simulink model "ROPOD_4Wheel_Tdistkinb_cntr_hosp_platform"  (R2017b)
settings: Solver=FixedStepAuto  StartTime=0.0  StopTime=Inf  FixedStep=Ts  RelTol=1e-3
PreLoadFcn:
  | init_model
InitFcn:
  | init_model
values from neighbouring files (symbols this model uses):
  FFtheta_intia = 0    [init_model.m]
  FFxy_mass = 0*80    (= 0)    [init_model.m]
  max_hw_tau = 7.0    (= 7)    [init_model.m]
  max_ropod_sw_force = 500    [init_model.m]
  max_ropod_sw_tau = 250    [init_model.m]
  Nwheels = 4    [Jqwl_numeric_function.m]    (also in S_matrix.m; extract_kinmodel_parameters.m; init_model.m; tau_optimal_dist_vec_fun.m)
  pivot_offs_sws = [2.663 3.74064 5.877 3.875]    [init_model.m]
  SW_COM1_ENABLE1 = hex2dec('0001')    [init_model.m]
  SW_COM1_ENABLE2 = hex2dec('0002')    [init_model.m]
  SW_COM1_MODE_TORQUE = bitshift(hex2dec('0000'),2)    [init_model.m]
  SW_COM1_MODE_VELOCITY = bitshift(hex2dec('0002'),2)    [init_model.m]
  SW_COM1_USE_TS = hex2dec('8000')    [init_model.m]
  sw_tau_2_curr = 1/motor_physical_parameters.torqueconstant.value    [init_model.m]
  Tinit = 5    [init_model.m]
  Ts = 0.001    [init_model.m]
  Tsp = 1    [init_model.m]
undefined symbols (not defined in the file or in its folder): DiscIntNeverNeededParam, Pose, ropod_kinmodel_param, Twist
libraries: robotlib x48, simulink x34, cstblocks x11, SOEM_EtherCAT_Lib x5, robotcorelib x1
(part 1 of 4)
PreSaveFcn:
  | init_model
settings Model: Creator=cesar  LastModifiedBy=cesar
settings OptimizationCC: PassReuseOutputArgsAs=Individual arguments  MaxStackSize=64
settings DebuggingCC: ParameterTunabilityLossMsg=error
settings HardwareCC: ProdBitPerLong=64  ProdHWDeviceType=Intel->x86-64 (Linux 64)  TargetBitPerLong=64  TargetBitPerPointer=64  TargetBitPerSizeT=64  TargetBitPerPtrDiffT=64  TargetLargestAtomicFloat=Float  TargetIntDivRoundTo=Zero  TargetEndianess=LittleEndian  TargetWordSize=64  TargetHWDeviceType=Intel->x86-64 (Linux 64)
settings SFSimCC: MATLABDynamicMemAlloc=off
settings RTWCC: SystemTargetFile=ert.tlc  HardwareBoard=Robot Operating System (ROS)  TemplateMakefile=ert_default_tmf  GenerateReport=on  RTWVerbose=off  CustomInclude=/usr/local/include/soem  CustomLibrary=/usr/local/lib/libsoem.so  Toolchain=Catkin  BuildConfiguration=Faster Runs  IncludeHyperlinkInReport=on  LaunchReport=on  TargetLang=C++  GenerateTraceInfo=on  GenerateTraceReport=on  GenerateTraceReportSl=on  GenerateTraceReportSf=on  GenerateTraceReportEml=on
settings CodeAppCC: ForceParamTrailComments=on  IgnoreCustomStorageClasses=off  OperatorAnnotations=on  SimulinkDataObjDesc=on  SFDataObjDesc=on  InsertBlockDesc=on
settings ERTTargetCC: SupportNonInlinedSFcns=on  SupportVariableSizeSignals=on

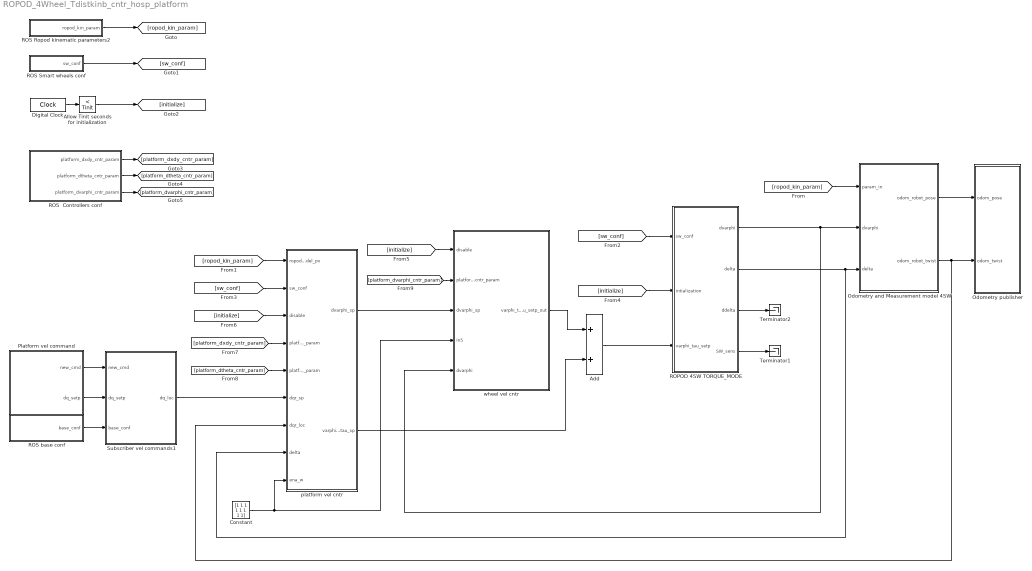
== system ROPOD_4Wheel_Tdistkinb_cntr_hosp_platform ==
  Add : Sum
  Allow Tinit seconds for initialization : simulink/Logic and Bit Operations/Compare To Constant  relop=<  const=Tinit  OutDataTypeStr=boolean
  Constant : Constant  Value=[1 1 1 1 1 1 1 1]
  Digital Clock : DigitalClock  SampleTime=Ts
  Odometry and Measurement model 4SW : Subsystem
  Odometry publisher : Subsystem
  Platform vel command : Subsystem
  ROPOD 4SW TORQUE_MODE : Subsystem
  ROS  Controllers conf : Subsystem
  ROS Ropod kinematic parameters2 : Subsystem
  ROS Smart wheels conf : Subsystem
  ROS base conf : Subsystem
  Subscriber vel commands1 : Subsystem
  Terminator1 : Terminator
  Terminator2 : Terminator
  platform vel cntr : Subsystem
  wheel vel cntr : Subsystem
  wires:
  Platform vel command/2(dq_setp) -> Subscriber vel commands1/2(dq_setp)
  ROS base conf/1(base_conf) -> Subscriber vel commands1/3(base_conf)
  ROPOD 4SW TORQUE_MODE/3(ddelta) -> Terminator2/1
  Add/1 -> ROPOD 4SW TORQUE_MODE/3(varphi_tau_setp)
  Constant/1 -> platform vel cntr/9(ena_w), wheel vel cntr/4(In5)
  Odometry and Measurement model 4SW/2(odom_robot_twist) -> platform vel cntr/7(dqr_loc), Odometry publisher/2(odom_twist)
  ROPOD 4SW TORQUE_MODE/4(SW_sens) -> Terminator1/1
  platform vel cntr/2(varphi_tau_sp) -> Add/2
  platform vel cntr/1(dvarphi_sp) -> wheel vel cntr/3(dvarphi_sp)
  ROPOD 4SW TORQUE_MODE/2(delta) -> platform vel cntr/8(delta), Odometry and Measurement model 4SW/3(delta)
  Digital Clock/1 -> Allow Tinit seconds for initialization/1
  ROS Ropod kinematic parameters2/1(ropod_kin_param) -> [ropod_kin_param]
  ROPOD 4SW TORQUE_MODE/1(dvarphi) -> Odometry and Measurement model 4SW/2(dvarphi), wheel vel cntr/5(dvarphi)
  ROS Smart wheels conf/1(sw_conf) -> [sw_conf]
  wheel vel cntr/1(varphi_tau_setp_out) -> Add/1
  Odometry and Measurement model 4SW/1(odom_robot_pose) -> Odometry publisher/1(odom_pose)
  Subscriber vel commands1/1(dq_loc) -> platform vel cntr/6(dqr_sp)
  [ropod_kin_param] -> Odometry and Measurement model 4SW/1(param_in)
  [ropod_kin_param] -> platform vel cntr/1(ropod_kinmodel_pv)
  [sw_conf] -> ROPOD 4SW TORQUE_MODE/1(sw_conf)
  [sw_conf] -> platform vel cntr/2(sw_conf)
  Allow Tinit seconds for initialization/1 -> [initialize]
  [initialize] -> ROPOD 4SW TORQUE_MODE/2(intialization)
  [initialize] -> wheel vel cntr/1(disable)
  [initialize] -> platform vel cntr/3(disable)
  ROS  Controllers conf/1(platform_dxdy_cntr_param) -> [platform_dxdy_cntr_param]
  ROS  Controllers conf/2(platform_dtheta_cntr_param) -> [platform_dtheta_cntr_param]
  ROS  Controllers conf/3(platform_dvarphi_cntr_param) -> [platform_dvarphi_cntr_param]
  [platform_dxdy_cntr_param] -> platform vel cntr/4(platform_dxdy_cntr_param)
  [platform_dtheta_cntr_param] -> platform vel cntr/5(platform_dtheta_cntr_param)
  [platform_dvarphi_cntr_param] -> wheel vel cntr/2(platform_dxdy_cntr_param)
  Platform vel command/1(new_cmd) -> Subscriber vel commands1/1(new_cmd)

== system ROPOD_4Wheel_Tdistkinb_cntr_hosp_platform/Odometry and Measurement model 4SW ==
  note: This output is only useful when using ros
      | This data is fed to /odom/pose
  note: This part is in global coordinates
  note: This part is in local coordinates
  param_in : Inport
  dvarphi : Inport  Port=2
  delta : Inport  Port=3
  Discrete-Time Integrator : DiscreteIntegrator  InitialConditionSetting=State (most efficient)  SampleTime=Ts  ICPrevOutput=DiscIntNeverNeededParam  ICPrevScaledInput=DiscIntNeverNeededParam
  Jqwl_matrix : MATLAB Function  TreatAsAtomicUnit=on
  Product3 : Product  Multiplication=Matrix(*)
  Selector3 : Selector  InputPortWidth=3  IndexOptions=Index vector (dialog)  Indices=3  OutputSizes=1
  Signal Specification : SignalSpecification  Dimensions=[3 1]
  pos_rot_matrix : MATLAB Function  TreatAsAtomicUnit=on
  odom_robot_pose : Outport
  odom_robot_twist : Outport  Port=2
  wires:
  Product3/1 -> Signal Specification/1
  param_in/1 -> Jqwl_matrix/1(ropod_kinmodel_param_vec)
  delta/1 -> Jqwl_matrix/2(delta)
  Jqwl_matrix/1(Jqwl) -> Product3/1
  dvarphi/1 -> Product3/2
  Signal Specification/1 -> pos_rot_matrix/1(dqr_loc), odom_robot_twist/1
  Selector3/1 -> pos_rot_matrix/2(theta_odom)
  pos_rot_matrix/1(dqr_glb) -> Discrete-Time Integrator/1
  Discrete-Time Integrator/1 -> odom_robot_pose/1, Selector3/1

== system ROPOD_4Wheel_Tdistkinb_cntr_hosp_platform/Odometry publisher ==
  odom_pose : Inport
  odom_twist : Inport  Port=2
  Blank Message : robotlib/Blank Message  SourceLibraryInfo=This block requires Robotics System Toolbox  messageType=nav_msgs/Odometry  SampleTime=-1
      settings: SourceProductBaseCode=RO
  Bus Assignment : BusAssignment  AssignedSignals=Pose.Pose.Position.X,Pose.Pose.Position.Y,Pose.Pose.Position.Z,Pose.Pose.Orientation.W,Pose.Pose.Orientation.X,Pose.Pose.Orientation.Y,Pose.Pose.Orientation.Z,Twist.Twist.Linear.X,Twist.Twist.Linear.Y,Twist.Twist.Linear.Z,Twist.Twist.Angular.X,Twist.Twist.Angular.Y,Twist.Twist.Angular.Z
  Constant{,1..5} (6 alike) : Constant  Value=0
  Coordinate Transformation Conversion : robotcorelib/Coordinate Transformation Conversion  InputRepresentation=Euler Angles  InputEulerSequence=XYZ  ShowTrVecInputPort=on  OutputRepresentation=Quaternion  OutputEulerSequence=ZYX  ShowTrVecOutputPort=on  SimulateUsing=Code generation
      settings: SourceProductBaseCode=RO
  Demux : Demux  Outputs=3
  Demux1 : Demux
  Demux2 : Demux  Outputs=3
  Mux : Mux  Inputs=3
  Publish : robotlib/Publish  SourceLibraryInfo=This block requires Robotics System Toolbox  topicSource=Specify your own  topic=/odom_incomplete  messageType=nav_msgs/Odometry  messageQueueLength=1
      settings: SourceProductBaseCode=RO
  Rate Transition : RateTransition  OutPortSampleTime=Ts_rost
  wires:
  Demux2/2 -> Bus Assignment/10
  Bus Assignment/1 -> Rate Transition/1
  Constant2/1 -> Mux/2
  Constant3/1 -> Bus Assignment/11
  Constant/1 -> Bus Assignment/4
  Constant4/1 -> Bus Assignment/12
  Demux2/1 -> Bus Assignment/9
  Coordinate Transformation Conversion/1 -> Demux1/1
  Constant5/1 -> Bus Assignment/13
  Demux/3 -> Mux/3
  Mux/1 -> Coordinate Transformation Conversion/1
  odom_pose/1 -> Demux/1
  Demux/1 -> Bus Assignment/2
  Constant1/1 -> Mux/1
  odom_twist/1 -> Demux2/1
  Demux/2 -> Bus Assignment/3
  Blank Message/1 -> Bus Assignment/1
  Demux2/3 -> Bus Assignment/14
  Rate Transition/1 -> Publish/1
  Demux1/1 -> Bus Assignment/5
  Demux1/2 -> Bus Assignment/6
  Demux1/3 -> Bus Assignment/7
  Demux1/4 -> Bus Assignment/8

== system ROPOD_4Wheel_Tdistkinb_cntr_hosp_platform/Platform vel command ==
  Subscribe1 : robotlib/Subscribe  SourceLibraryInfo=This block requires Robotics System Toolbox  topicSource=Specify your own  topic=/cmd_vel  messageType=geometry_msgs/Twist  sampleTime=Ts_rost  messageQueueLength=5
      settings: SourceProductBaseCode=RO
  new_cmd : Outport
  dq_setp : Outport  Port=2
  wires:
  Subscribe1/2 -> dq_setp/1
  Subscribe1/1 -> new_cmd/1

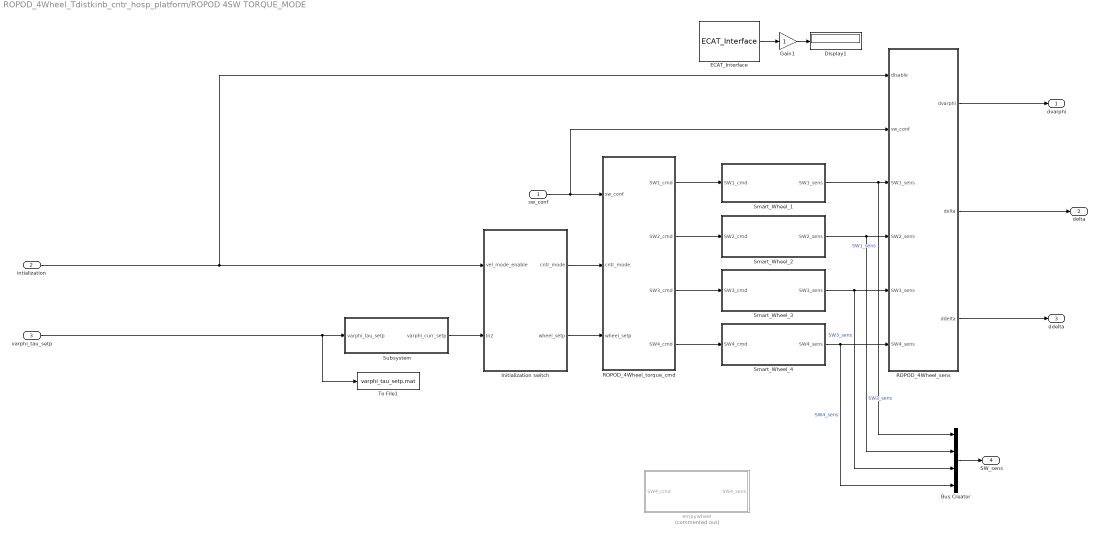
== system ROPOD_4Wheel_Tdistkinb_cntr_hosp_platform/ROPOD 4SW TORQUE_MODE ==
  sw_conf : Inport
  intialization : Inport  Port=2
  varphi_tau_setp : Inport  Port=3
  Bus Creator : BusCreator  Inputs=4
  Display1 : Display
  ECAT_Interface : SOEM_EtherCAT_Lib/ECAT_Interface  Priority=0  IFINTERFACE=eth0  TS=Ts
      settings: SourceProductName=SOEM_EtherCAT_Lib
  Gain1 : Gain  OutDataTypeStr=double
  Initialization switch : Subsystem
  ROPOD_4Wheel_sens : Subsystem
  ROPOD_4Wheel_torque_cmd : Subsystem
  Smart_Wheel_1 : Subsystem
  Smart_Wheel_2 : Subsystem
  Smart_Wheel_3 : Subsystem
  Smart_Wheel_4 : Subsystem
  Subsystem : Subsystem
  To File1 : ToFile  Filename=varphi_tau_setp.mat  MatrixName=varphi_tau_setp
  empywheel : Subsystem  Commented=on
  dvarphi : Outport
  delta : Outport  Port=2
  ddelta : Outport  Port=3
  SW_sens : Outport  Port=4
  wires:
  ROPOD_4Wheel_sens/2(delta) -> delta/1
  ROPOD_4Wheel_sens/1(dvarphi) -> dvarphi/1
  ECAT_Interface/1 -> Gain1/1
  Gain1/1 -> Display1/1
  ROPOD_4Wheel_sens/3(ddelta) -> ddelta/1
  ROPOD_4Wheel_torque_cmd/4(SW4_cmd) -> Smart_Wheel_4/1(SW4_cmd)
  ROPOD_4Wheel_torque_cmd/1(SW1_cmd) -> Smart_Wheel_1/1(SW1_cmd)
  ROPOD_4Wheel_torque_cmd/3(SW3_cmd) -> Smart_Wheel_3/1(SW3_cmd)
  sw_conf/1 -> ROPOD_4Wheel_torque_cmd/1(sw_conf), ROPOD_4Wheel_sens/2(sw_conf)
  ROPOD_4Wheel_torque_cmd/2(SW2_cmd) -> Smart_Wheel_2/1(SW2_cmd)
  Smart_Wheel_1/1(SW1_sens) -> Bus Creator/1, ROPOD_4Wheel_sens/3(SW1_sens)  "SW1_sens"
  Smart_Wheel_4/1(SW4_sens) -> ROPOD_4Wheel_sens/6(SW4_sens), Bus Creator/4  "SW4_sens"
  Smart_Wheel_2/1(SW2_sens) -> ROPOD_4Wheel_sens/4(SW2_sens), Bus Creator/2  "SW2_sens"
  Smart_Wheel_3/1(SW3_sens) -> ROPOD_4Wheel_sens/5(SW3_sens), Bus Creator/3  "SW3_sens"
  Bus Creator/1 -> SW_sens/1
  Initialization switch/1(cntr_mode) -> ROPOD_4Wheel_torque_cmd/2(cntr_mode)
  Initialization switch/2(wheel_setp) -> ROPOD_4Wheel_torque_cmd/3(wheel_setp)
  Subsystem/1(varphi_curr_setp) -> Initialization switch/2(In2)
  varphi_tau_setp/1 -> To File1/1, Subsystem/1(varphi_tau_setp)
  intialization/1 -> ROPOD_4Wheel_sens/1(disable), Initialization switch/1(vel_mode_enable)

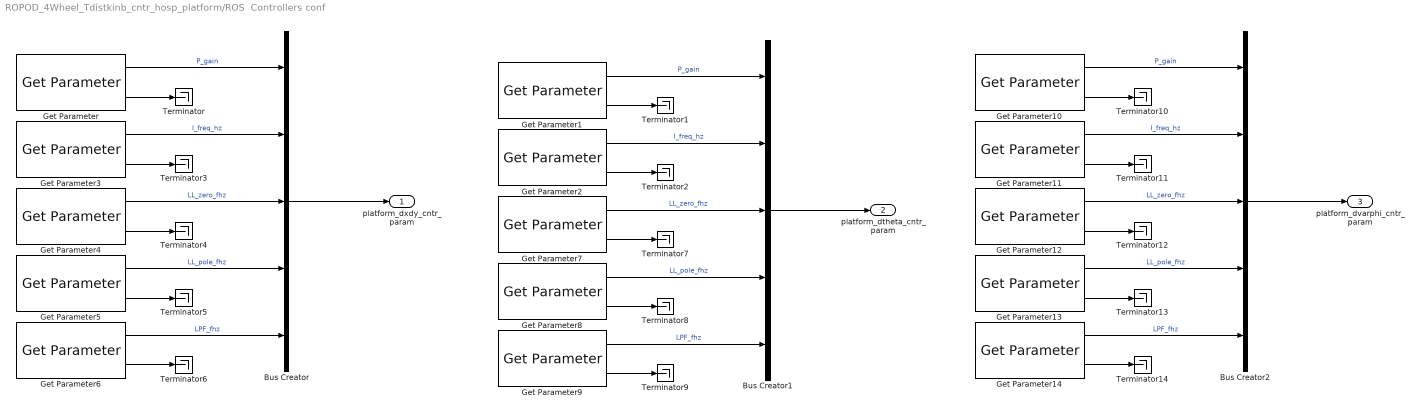
== system ROPOD_4Wheel_Tdistkinb_cntr_hosp_platform/ROS  Controllers conf ==
  Bus Creator : BusCreator  Inputs=5
  Bus Creator1 : BusCreator  Inputs=5
  Bus Creator2 : BusCreator  Inputs=5
  Get Parameter : robotlib/Get Parameter  SourceLibraryInfo=This block requires Robotics System Toolbox  ParameterSource=Specify your own  ParameterName=/ropod/ropod_4wheel_kinb_cntr_node/platform_dxdy_cntr/Kgain  ParameterType=double  ParameterMaxArrayLength=16  ParameterInitialValue=K_gain_dxdy_cntr  SampleTime=Tsp  ShowErrorCodeOutput=on  ModelName=ROPOD_4Wheel_Tdistkinb_cntr  BlockId=ParamGet_ROPOD_4Wheel_Tdistkinb_cntr_2716
      settings: SourceProductName=Robotics System Toolbox  SourceProductBaseCode=RO
  Get Parameter1 : robotlib/Get Parameter  SourceLibraryInfo=This block requires Robotics System Toolbox  ParameterSource=Specify your own  ParameterName=/ropod/ropod_4wheel_kinb_cntr_node/platform_dtheta_cntr/Kgain  ParameterType=double  ParameterMaxArrayLength=16  ParameterInitialValue=K_gain_dtheta_cntr  SampleTime=Tsp  ShowErrorCodeOutput=on  ModelName=ROPOD_4Wheel_Tdistkinb_cntr  BlockId=ParamGet_ROPOD_4Wheel_Tdistkinb_cntr_2919
      settings: SourceProductName=Robotics System Toolbox  SourceProductBaseCode=RO
  Get Parameter10 : robotlib/Get Parameter  SourceLibraryInfo=This block requires Robotics System Toolbox  ParameterSource=Specify your own  ParameterName=/ropod/ropod_4wheel_kinb_cntr_node/platform_dvarphi_cntr/Kgain  ParameterType=double  ParameterMaxArrayLength=16  ParameterInitialValue=K_gain_dvarphi_cntr  SampleTime=Tsp  ShowErrorCodeOutput=on  ModelName=ROPOD_4Wheel_Tdistkinb_cntr  BlockId=ParamGet_ROPOD_4Wheel_Tdistkinb_cntr_2931
      settings: SourceProductName=Robotics System Toolbox  SourceProductBaseCode=RO
  Get Parameter11 : robotlib/Get Parameter  SourceLibraryInfo=This block requires Robotics System Toolbox  ParameterSource=Specify your own  ParameterName=/ropod/ropod_4wheel_kinb_cntr_node/platform_dvarphi_cntr/I_fhz  ParameterType=double  ParameterMaxArrayLength=16  ParameterInitialValue=I_fhz_dvarphi_cntr  SampleTime=Tsp  ShowErrorCodeOutput=on  ModelName=ROPOD_4Wheel_Tdistkinb_cntr  BlockId=ParamGet_ROPOD_4Wheel_Tdistkinb_cntr_2932
      settings: SourceProductName=Robotics System Toolbox  SourceProductBaseCode=RO
  Get Parameter12 : robotlib/Get Parameter  SourceLibraryInfo=This block requires Robotics System Toolbox  ParameterSource=Specify your own  ParameterName=/ropod/ropod_4wheel_kinb_cntr_node/platform_dvarphi_cntr/LL_wz_fhz  ParameterType=double  ParameterMaxArrayLength=16  ParameterInitialValue=LL_wz_fhz_dvarphi_cntr  SampleTime=Tsp  ShowErrorCodeOutput=on  ModelName=ROPOD_4Wheel_Tdistkinb_cntr  BlockId=ParamGet_ROPOD_4Wheel_Tdistkinb_cntr_2933
      settings: SourceProductName=Robotics System Toolbox  SourceProductBaseCode=RO
  Get Parameter13 : robotlib/Get Parameter  SourceLibraryInfo=This block requires Robotics System Toolbox  ParameterSource=Specify your own  ParameterName=/ropod/ropod_4wheel_kinb_cntr_node/platform_dvarphi_cntr/LL_wp_fhz  ParameterType=double  ParameterMaxArrayLength=16  ParameterInitialValue=LL_wp_fhz_dvarphi_cntr  SampleTime=Tsp  ShowErrorCodeOutput=on  ModelName=ROPOD_4Wheel_Tdistkinb_cntr  BlockId=ParamGet_ROPOD_4Wheel_Tdistkinb_cntr_2934
      settings: SourceProductName=Robotics System Toolbox  SourceProductBaseCode=RO
  Get Parameter14 : robotlib/Get Parameter  SourceLibraryInfo=This block requires Robotics System Toolbox  ParameterSource=Specify your own  ParameterName=/ropod/ropod_4wheel_kinb_cntr_node/platform_dvarphi_cntr/LPF_fhz  ParameterType=double  ParameterMaxArrayLength=16  ParameterInitialValue=LPF_fhz_dvarphi_cntr  SampleTime=Tsp  ShowErrorCodeOutput=on  ModelName=ROPOD_4Wheel_Tdistkinb_cntr  BlockId=ParamGet_ROPOD_4Wheel_Tdistkinb_cntr_2935
      settings: SourceProductName=Robotics System Toolbox  SourceProductBaseCode=RO
  Get Parameter2 : robotlib/Get Parameter  SourceLibraryInfo=This block requires Robotics System Toolbox  ParameterSource=Specify your own  ParameterName=/ropod/ropod_4wheel_kinb_cntr_node/platform_dtheta_cntr/I_fhz  ParameterType=double  ParameterMaxArrayLength=16  ParameterInitialValue=I_fhz_dtheta_cntr  SampleTime=Tsp  ShowErrorCodeOutput=on  ModelName=ROPOD_4Wheel_Tdistkinb_cntr  BlockId=ParamGet_ROPOD_4Wheel_Tdistkinb_cntr_2920
      settings: SourceProductName=Robotics System Toolbox  SourceProductBaseCode=RO
  Get Parameter3 : robotlib/Get Parameter  SourceLibraryInfo=This block requires Robotics System Toolbox  ParameterSource=Specify your own  ParameterName=/ropod/ropod_4wheel_kinb_cntr_node/platform_dxdy_cntr/I_fhz  ParameterType=double  ParameterMaxArrayLength=16  ParameterInitialValue=I_fhz_dxdy_cntr  SampleTime=Tsp  ShowErrorCodeOutput=on  ModelName=ROPOD_4Wheel_Tdistkinb_cntr  BlockId=ParamGet_ROPOD_4Wheel_Tdistkinb_cntr_2898
      settings: SourceProductName=Robotics System Toolbox  SourceProductBaseCode=RO
  Get Parameter4 : robotlib/Get Parameter  SourceLibraryInfo=This block requires Robotics System Toolbox  ParameterSource=Specify your own  ParameterName=/ropod/ropod_4wheel_kinb_cntr_node/platform_dxdy_cntr/LL_wz_fhz  ParameterType=double  ParameterMaxArrayLength=16  ParameterInitialValue=LL_wz_fhz_dxdy_cntr  SampleTime=Tsp  ShowErrorCodeOutput=on  ModelName=ROPOD_4Wheel_Tdistkinb_cntr  BlockId=ParamGet_ROPOD_4Wheel_Tdistkinb_cntr_2900
      settings: SourceProductName=Robotics System Toolbox  SourceProductBaseCode=RO
  Get Parameter5 : robotlib/Get Parameter  SourceLibraryInfo=This block requires Robotics System Toolbox  ParameterSource=Specify your own  ParameterName=/ropod/ropod_4wheel_kinb_cntr_node/platform_dxdy_cntr/LL_wp_fhz  ParameterType=double  ParameterMaxArrayLength=16  ParameterInitialValue=LL_wp_fhz_dxdy_cntr  SampleTime=Tsp  ShowErrorCodeOutput=on  ModelName=ROPOD_4Wheel_Tdistkinb_cntr  BlockId=ParamGet_ROPOD_4Wheel_Tdistkinb_cntr_2902
      settings: SourceProductName=Robotics System Toolbox  SourceProductBaseCode=RO
  Get Parameter6 : robotlib/Get Parameter  SourceLibraryInfo=This block requires Robotics System Toolbox  ParameterSource=Specify your own  ParameterName=/ropod/ropod_4wheel_kinb_cntr_node/platform_dxdy_cntr/LPF_fhz  ParameterType=double  ParameterMaxArrayLength=16  ParameterInitialValue=LPF_fhz_dxdy_cntr  SampleTime=Tsp  ShowErrorCodeOutput=on  ModelName=ROPOD_4Wheel_Tdistkinb_cntr  BlockId=ParamGet_ROPOD_4Wheel_Tdistkinb_cntr_2903
      settings: SourceProductName=Robotics System Toolbox  SourceProductBaseCode=RO
  Get Parameter7 : robotlib/Get Parameter  SourceLibraryInfo=This block requires Robotics System Toolbox  ParameterSource=Specify your own  ParameterName=/ropod/ropod_4wheel_kinb_cntr_node/platform_dtheta_cntr/LL_wz_fhz  ParameterType=double  ParameterMaxArrayLength=16  ParameterInitialValue=LL_wz_fhz_dtheta_cntr  SampleTime=Tsp  ShowErrorCodeOutput=on  ModelName=ROPOD_4Wheel_Tdistkinb_cntr  BlockId=ParamGet_ROPOD_4Wheel_Tdistkinb_cntr_2921
      settings: SourceProductName=Robotics System Toolbox  SourceProductBaseCode=RO
  Get Parameter8 : robotlib/Get Parameter  SourceLibraryInfo=This block requires Robotics System Toolbox  ParameterSource=Specify your own  ParameterName=/ropod/ropod_4wheel_kinb_cntr_node/platform_dtheta_cntr/LL_wp_fhz  ParameterType=double  ParameterMaxArrayLength=16  ParameterInitialValue=LL_wp_fhz_dtheta_cntr  SampleTime=Tsp  ShowErrorCodeOutput=on  ModelName=ROPOD_4Wheel_Tdistkinb_cntr  BlockId=ParamGet_ROPOD_4Wheel_Tdistkinb_cntr_2922
      settings: SourceProductName=Robotics System Toolbox  SourceProductBaseCode=RO
  Get Parameter9 : robotlib/Get Parameter  SourceLibraryInfo=This block requires Robotics System Toolbox  ParameterSource=Specify your own  ParameterName=/ropod/ropod_4wheel_kinb_cntr_node/platform_dtheta_cntr/LPF_fhz  ParameterType=double  ParameterMaxArrayLength=16  ParameterInitialValue=LPF_fhz_dtheta_cntr  SampleTime=Tsp  ShowErrorCodeOutput=on  ModelName=ROPOD_4Wheel_Tdistkinb_cntr  BlockId=ParamGet_ROPOD_4Wheel_Tdistkinb_cntr_2923
      settings: SourceProductName=Robotics System Toolbox  SourceProductBaseCode=RO
  Terminator{,1..14} (15 alike) : Terminator
  platform_dxdy_cntr_param : Outport
  platform_dtheta_cntr_param : Outport  Port=2
  platform_dvarphi_cntr_param : Outport  Port=3
  wires:
  Get Parameter/2 -> Terminator/1
  Get Parameter5/1 -> Bus Creator/4  "LL_pole_fhz"
  Get Parameter6/1 -> Bus Creator/5  "LPF_fhz"
  Bus Creator/1 -> platform_dxdy_cntr_param/1
  Get Parameter3/1 -> Bus Creator/2  "I_freq_hz"
  Get Parameter4/1 -> Bus Creator/3  "LL_zero_fhz"
  Get Parameter/1 -> Bus Creator/1  "P_gain"
  Get Parameter3/2 -> Terminator3/1
  Get Parameter4/2 -> Terminator4/1
  Get Parameter5/2 -> Terminator5/1
  Get Parameter6/2 -> Terminator6/1
  Get Parameter8/1 -> Bus Creator1/4  "LL_pole_fhz"
  Get Parameter9/2 -> Terminator9/1
  Get Parameter2/1 -> Bus Creator1/2  "I_freq_hz"
  Get Parameter8/2 -> Terminator8/1
  Bus Creator1/1 -> platform_dtheta_cntr_param/1
  Get Parameter2/2 -> Terminator2/1
  Get Parameter7/1 -> Bus Creator1/3  "LL_zero_fhz"
  Get Parameter7/2 -> Terminator7/1
  Get Parameter1/1 -> Bus Creator1/1  "P_gain"
  Get Parameter1/2 -> Terminator1/1
  Get Parameter9/1 -> Bus Creator1/5  "LPF_fhz"
  Get Parameter10/2 -> Terminator10/1
  Get Parameter13/2 -> Terminator13/1
  Get Parameter14/2 -> Terminator14/1
  Get Parameter11/1 -> Bus Creator2/2  "I_freq_hz"
  Get Parameter10/1 -> Bus Creator2/1  "P_gain"
  Get Parameter11/2 -> Terminator11/1
  Get Parameter13/1 -> Bus Creator2/4  "LL_pole_fhz"
  Bus Creator2/1 -> platform_dvarphi_cntr_param/1
  Get Parameter12/2 -> Terminator12/1
  Get Parameter12/1 -> Bus Creator2/3  "LL_zero_fhz"
  Get Parameter14/1 -> Bus Creator2/5  "LPF_fhz"

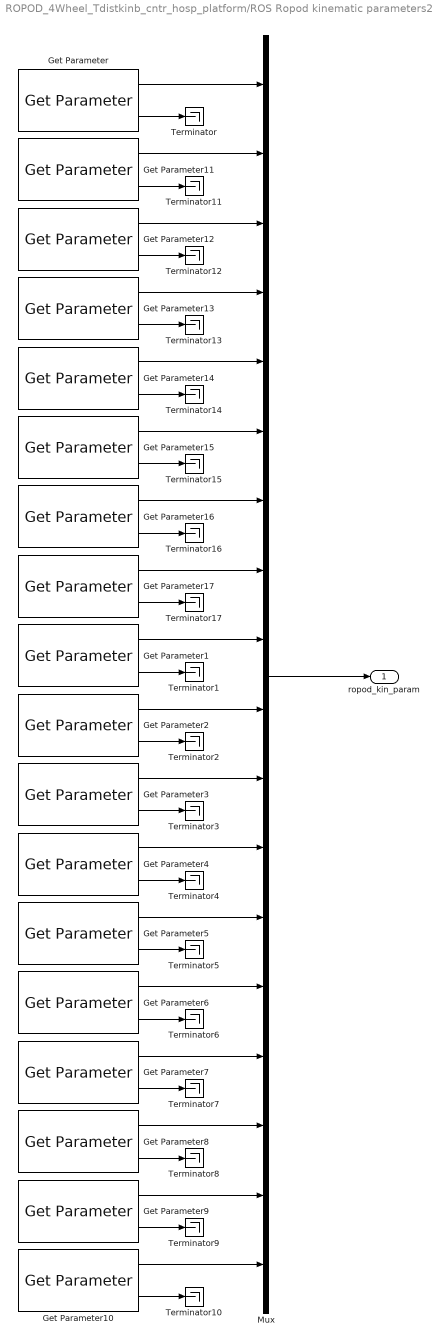
== system ROPOD_4Wheel_Tdistkinb_cntr_hosp_platform/ROS Ropod kinematic parameters2 ==
  Get Parameter : robotlib/Get Parameter  SourceLibraryInfo=This block requires Robotics System Toolbox  ParameterSource=Specify your own  ParameterName=/ropod/ropod_4wheel_kinb_cntr_node/base_kin_model/r_wL_SW1  ParameterType=double  ParameterMaxArrayLength=16  ParameterInitialValue=ropod_kinmodel_param.r_w(1)  SampleTime=Tsp  ShowErrorCodeOutput=on  ModelName=ROPOD_4Wheel_Tdistkinb_cntr  BlockId=ParamGet_ROPOD_4Wheel_Tdistkinb_cntr_2173
      settings: SourceProductName=Robotics System Toolbox  SourceProductBaseCode=RO
  Get Parameter1 : robotlib/Get Parameter  SourceLibraryInfo=This block requires Robotics System Toolbox  ParameterSource=Specify your own  ParameterName=/ropod/ropod_4wheel_kinb_cntr_node/base_kin_model/s_w  ParameterType=double  ParameterMaxArrayLength=16  ParameterInitialValue=ropod_kinmodel_param.s_w  SampleTime=Tsp  ShowErrorCodeOutput=on  ModelName=ROPOD_4Wheel_Tdistkinb_cntr  BlockId=ParamGet_ROPOD_4Wheel_Tdistkinb_cntr_2174
      settings: SourceProductName=Robotics System Toolbox  SourceProductBaseCode=RO
  Get Parameter10 : robotlib/Get Parameter  SourceLibraryInfo=This block requires Robotics System Toolbox  ParameterSource=Specify your own  ParameterName=/ropod/ropod_4wheel_kinb_cntr_node/base_kin_model/ypos_SW4  ParameterType=double  ParameterMaxArrayLength=16  ParameterInitialValue=ropod_kinmodel_param.C_SW(8)  SampleTime=Tsp  ShowErrorCodeOutput=on  ModelName=ROPOD_4Wheel_Tdistkinb_cntr  BlockId=ParamGet_ROPOD_4Wheel_Tdistkinb_cntr_2175
      settings: SourceProductName=Robotics System Toolbox  SourceProductBaseCode=RO
  Get Parameter11 : robotlib/Get Parameter  SourceLibraryInfo=This block requires Robotics System Toolbox  ParameterSource=Specify your own  ParameterName=/ropod/ropod_4wheel_kinb_cntr_node/base_kin_model/r_wR_SW1  ParameterType=double  ParameterMaxArrayLength=16  ParameterInitialValue=ropod_kinmodel_param.r_w(2)  SampleTime=Tsp  ShowErrorCodeOutput=on  ModelName=ROPOD_4Wheel_Tdistkinb_cntr  BlockId=ParamGet_ROPOD_4Wheel_Tdistkinb_cntr_2176
      settings: SourceProductName=Robotics System Toolbox  SourceProductBaseCode=RO
  Get Parameter12 : robotlib/Get Parameter  SourceLibraryInfo=This block requires Robotics System Toolbox  ParameterSource=Specify your own  ParameterName=/ropod/ropod_4wheel_kinb_cntr_node/base_kin_model/r_wL_SW2  ParameterType=double  ParameterMaxArrayLength=16  ParameterInitialValue=ropod_kinmodel_param.r_w(3)  SampleTime=Tsp  ShowErrorCodeOutput=on  ModelName=ROPOD_4Wheel_Tdistkinb_cntr  BlockId=ParamGet_ROPOD_4Wheel_Tdistkinb_cntr_2177
      settings: SourceProductName=Robotics System Toolbox  SourceProductBaseCode=RO
  Get Parameter13 : robotlib/Get Parameter  SourceLibraryInfo=This block requires Robotics System Toolbox  ParameterSource=Specify your own  ParameterName=/ropod/ropod_4wheel_kinb_cntr_node/base_kin_model/r_wR_SW2  ParameterType=double  ParameterMaxArrayLength=16  ParameterInitialValue=ropod_kinmodel_param.r_w(4)  SampleTime=Tsp  ShowErrorCodeOutput=on  ModelName=ROPOD_4Wheel_Tdistkinb_cntr  BlockId=ParamGet_ROPOD_4Wheel_Tdistkinb_cntr_2178
      settings: SourceProductName=Robotics System Toolbox  SourceProductBaseCode=RO
  Get Parameter14 : robotlib/Get Parameter  SourceLibraryInfo=This block requires Robotics System Toolbox  ParameterSource=Specify your own  ParameterName=/ropod/ropod_4wheel_kinb_cntr_node/base_kin_model/r_wL_SW3  ParameterType=double  ParameterMaxArrayLength=16  ParameterInitialValue=ropod_kinmodel_param.r_w(5)  SampleTime=Tsp  ShowErrorCodeOutput=on  ModelName=ROPOD_4Wheel_Tdistkinb_cntr  BlockId=ParamGet_ROPOD_4Wheel_Tdistkinb_cntr_2179
      settings: SourceProductName=Robotics System Toolbox  SourceProductBaseCode=RO
  Get Parameter15 : robotlib/Get Parameter  SourceLibraryInfo=This block requires Robotics System Toolbox  ParameterSource=Specify your own  ParameterName=/ropod/ropod_4wheel_kinb_cntr_node/base_kin_model/r_wR_SW3  ParameterType=double  ParameterMaxArrayLength=16  ParameterInitialValue=ropod_kinmodel_param.r_w(6)  SampleTime=Tsp  ShowErrorCodeOutput=on  ModelName=ROPOD_4Wheel_Tdistkinb_cntr  BlockId=ParamGet_ROPOD_4Wheel_Tdistkinb_cntr_2180
      settings: SourceProductName=Robotics System Toolbox  SourceProductBaseCode=RO
  Get Parameter16 : robotlib/Get Parameter  SourceLibraryInfo=This block requires Robotics System Toolbox  ParameterSource=Specify your own  ParameterName=/ropod/ropod_4wheel_kinb_cntr_node/base_kin_model/r_wL_SW4  ParameterType=double  ParameterMaxArrayLength=16  ParameterInitialValue=ropod_kinmodel_param.r_w(7)  SampleTime=Tsp  ShowErrorCodeOutput=on  ModelName=ROPOD_4Wheel_Tdistkinb_cntr  BlockId=ParamGet_ROPOD_4Wheel_Tdistkinb_cntr_2181
      settings: SourceProductName=Robotics System Toolbox  SourceProductBaseCode=RO
  Get Parameter17 : robotlib/Get Parameter  SourceLibraryInfo=This block requires Robotics System Toolbox  ParameterSource=Specify your own  ParameterName=/ropod/ropod_4wheel_kinb_cntr_node/base_kin_model/r_wR_SW4  ParameterType=double  ParameterMaxArrayLength=16  ParameterInitialValue=ropod_kinmodel_param.r_w(8)  SampleTime=Tsp  ShowErrorCodeOutput=on  ModelName=ROPOD_4Wheel_Tdistkinb_cntr  BlockId=ParamGet_ROPOD_4Wheel_Tdistkinb_cntr_2182
      settings: SourceProductName=Robotics System Toolbox  SourceProductBaseCode=RO
  Get Parameter2 : robotlib/Get Parameter  SourceLibraryInfo=This block requires Robotics System Toolbox  ParameterSource=Specify your own  ParameterName=/ropod/ropod_4wheel_kinb_cntr_node/base_kin_model/d_w  ParameterType=double  ParameterMaxArrayLength=16  ParameterInitialValue=ropod_kinmodel_param.d_w  SampleTime=Tsp  ShowErrorCodeOutput=on  ModelName=ROPOD_4Wheel_Tdistkinb_cntr  BlockId=ParamGet_ROPOD_4Wheel_Tdistkinb_cntr_2183
      settings: SourceProductName=Robotics System Toolbox  SourceProductBaseCode=RO
  Get Parameter3 : robotlib/Get Parameter  SourceLibraryInfo=This block requires Robotics System Toolbox  ParameterSource=Specify your own  ParameterName=/ropod/ropod_4wheel_kinb_cntr_node/base_kin_model/xpos_SW1  ParameterType=double  ParameterMaxArrayLength=16  ParameterInitialValue=ropod_kinmodel_param.C_SW(1)  SampleTime=Tsp  ShowErrorCodeOutput=on  ModelName=ROPOD_4Wheel_Tdistkinb_cntr  BlockId=ParamGet_ROPOD_4Wheel_Tdistkinb_cntr_2184
      settings: SourceProductName=Robotics System Toolbox  SourceProductBaseCode=RO
  Get Parameter4 : robotlib/Get Parameter  SourceLibraryInfo=This block requires Robotics System Toolbox  ParameterSource=Specify your own  ParameterName=/ropod/ropod_4wheel_kinb_cntr_node/base_kin_model/ypos_SW1  ParameterType=double  ParameterMaxArrayLength=16  ParameterInitialValue=ropod_kinmodel_param.C_SW(2)  SampleTime=Tsp  ShowErrorCodeOutput=on  ModelName=ROPOD_4Wheel_Tdistkinb_cntr  BlockId=ParamGet_ROPOD_4Wheel_Tdistkinb_cntr_2185
      settings: SourceProductName=Robotics System Toolbox  SourceProductBaseCode=RO
  Get Parameter5 : robotlib/Get Parameter  SourceLibraryInfo=This block requires Robotics System Toolbox  ParameterSource=Specify your own  ParameterName=/ropod/ropod_4wheel_kinb_cntr_node/base_kin_model/xpos_SW2  ParameterType=double  ParameterMaxArrayLength=16  ParameterInitialValue=ropod_kinmodel_param.C_SW(3)  SampleTime=Tsp  ShowErrorCodeOutput=on  ModelName=ROPOD_4Wheel_Tdistkinb_cntr  BlockId=ParamGet_ROPOD_4Wheel_Tdistkinb_cntr_2186
      settings: SourceProductName=Robotics System Toolbox  SourceProductBaseCode=RO
  Get Parameter6 : robotlib/Get Parameter  SourceLibraryInfo=This block requires Robotics System Toolbox  ParameterSource=Specify your own  ParameterName=/ropod/ropod_4wheel_kinb_cntr_node/base_kin_model/ypos_SW2  ParameterType=double  ParameterMaxArrayLength=16  ParameterInitialValue=ropod_kinmodel_param.C_SW(4)  SampleTime=Tsp  ShowErrorCodeOutput=on  ModelName=ROPOD_4Wheel_Tdistkinb_cntr  BlockId=ParamGet_ROPOD_4Wheel_Tdistkinb_cntr_2187
      settings: SourceProductName=Robotics System Toolbox  SourceProductBaseCode=RO
  Get Parameter7 : robotlib/Get Parameter  SourceLibraryInfo=This block requires Robotics System Toolbox  ParameterSource=Specify your own  ParameterName=/ropod/ropod_4wheel_kinb_cntr_node/base_kin_model/xpos_SW3  ParameterType=double  ParameterMaxArrayLength=16  ParameterInitialValue=ropod_kinmodel_param.C_SW(5)  SampleTime=Tsp  ShowErrorCodeOutput=on  ModelName=ROPOD_4Wheel_Tdistkinb_cntr  BlockId=ParamGet_ROPOD_4Wheel_Tdistkinb_cntr_2188
      settings: SourceProductName=Robotics System Toolbox  SourceProductBaseCode=RO
  Get Parameter8 : robotlib/Get Parameter  SourceLibraryInfo=This block requires Robotics System Toolbox  ParameterSource=Specify your own  ParameterName=/ropod/ropod_4wheel_kinb_cntr_node/base_kin_model/ypos_SW3  ParameterType=double  ParameterMaxArrayLength=16  ParameterInitialValue=ropod_kinmodel_param.C_SW(6)  SampleTime=Tsp  ShowErrorCodeOutput=on  ModelName=ROPOD_4Wheel_Tdistkinb_cntr  BlockId=ParamGet_ROPOD_4Wheel_Tdistkinb_cntr_2189
      settings: SourceProductName=Robotics System Toolbox  SourceProductBaseCode=RO
  Get Parameter9 : robotlib/Get Parameter  SourceLibraryInfo=This block requires Robotics System Toolbox  ParameterSource=Specify your own  ParameterName=/ropod/ropod_4wheel_kinb_cntr_node/base_kin_model/xpos_SW4  ParameterType=double  ParameterMaxArrayLength=16  ParameterInitialValue=ropod_kinmodel_param.C_SW(7)  SampleTime=Tsp  ShowErrorCodeOutput=on  ModelName=ROPOD_4Wheel_Tdistkinb_cntr  BlockId=ParamGet_ROPOD_4Wheel_Tdistkinb_cntr_2190
      settings: SourceProductName=Robotics System Toolbox  SourceProductBaseCode=RO
  Mux : Mux  Inputs=18
  Terminator{,1..17} (18 alike) : Terminator
  ropod_kin_param : Outport
  wires:
  Mux/1 -> ropod_kin_param/1
  Get Parameter/2 -> Terminator/1
  Get Parameter13/1 -> Mux/4
  Get Parameter15/2 -> Terminator15/1
  Get Parameter14/2 -> Terminator14/1
  Get Parameter16/1 -> Mux/7
  Get Parameter15/1 -> Mux/6
  Get Parameter11/1 -> Mux/2
  Get Parameter11/2 -> Terminator11/1
  Get Parameter16/2 -> Terminator16/1
  Get Parameter12/2 -> Terminator12/1
  Get Parameter12/1 -> Mux/3
  Get Parameter/1 -> Mux/1
  Get Parameter17/2 -> Terminator17/1
  Get Parameter13/2 -> Terminator13/1
  Get Parameter17/1 -> Mux/8
  Get Parameter14/1 -> Mux/5
  Get Parameter2/2 -> Terminator2/1
  Get Parameter2/1 -> Mux/10
  Get Parameter1/1 -> Mux/9
  Get Parameter1/2 -> Terminator1/1
  Get Parameter6/2 -> Terminator6/1
  Get Parameter6/1 -> Mux/14
  Get Parameter3/1 -> Mux/11
  Get Parameter5/2 -> Terminator5/1
  Get Parameter5/1 -> Mux/13
  Get Parameter4/1 -> Mux/12
  Get Parameter3/2 -> Terminator3/1
  Get Parameter4/2 -> Terminator4/1
  Get Parameter10/1 -> Mux/18
  Get Parameter10/2 -> Terminator10/1
  Get Parameter8/2 -> Terminator8/1
  Get Parameter7/2 -> Terminator7/1
  Get Parameter9/2 -> Terminator9/1
  Get Parameter7/1 -> Mux/15
  Get Parameter8/1 -> Mux/16
  Get Parameter9/1 -> Mux/17

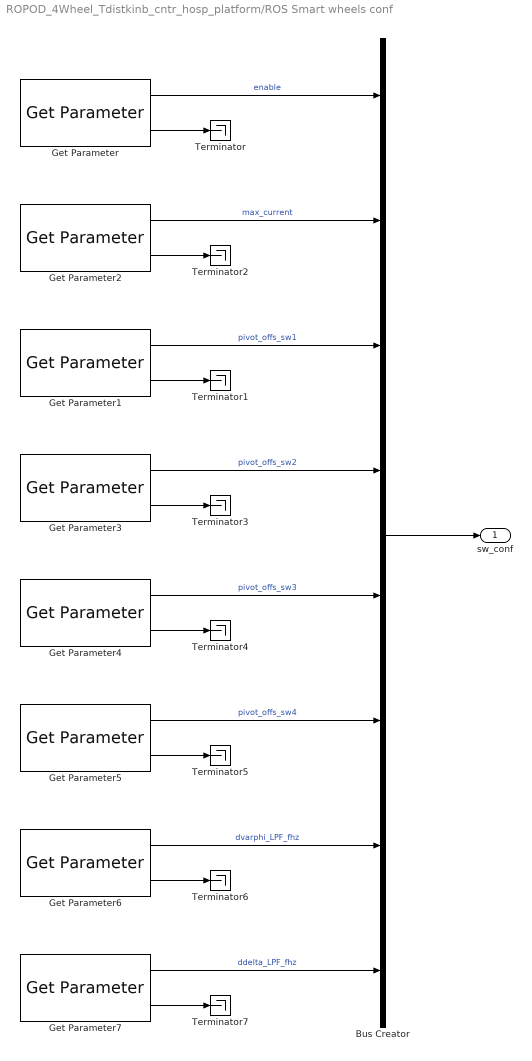
== system ROPOD_4Wheel_Tdistkinb_cntr_hosp_platform/ROS Smart wheels conf ==
  Bus Creator : BusCreator  Inputs=8
  Get Parameter : robotlib/Get Parameter  SourceLibraryInfo=This block requires Robotics System Toolbox  ParameterSource=Specify your own  ParameterName=/ropod/ropod_4wheel_kinb_cntr_node/smart_wheels/enable  ParameterType=double  ParameterMaxArrayLength=16  ParameterInitialValue=sw_ini_enable  SampleTime=Tsp  ShowErrorCodeOutput=on  ModelName=ROPOD_4Wheel_Tdistkinb_cntr  BlockId=ParamGet_ROPOD_4Wheel_Tdistkinb_cntr_2213
      settings: SourceProductName=Robotics System Toolbox  SourceProductBaseCode=RO
  Get Parameter1 : robotlib/Get Parameter  SourceLibraryInfo=This block requires Robotics System Toolbox  ParameterSource=Specify your own  ParameterName=/ropod/ropod_4wheel_kinb_cntr_node/smart_wheels/pivot_offs_sw1  ParameterType=double  ParameterMaxArrayLength=16  ParameterInitialValue=pivot_offs_sws(1)  SampleTime=Tsp  ShowErrorCodeOutput=on  ModelName=ROPOD_4Wheel_Tdistkinb_cntr  BlockId=ParamGet_ROPOD_4Wheel_Tdistkinb_cntr_2214
      settings: SourceProductName=Robotics System Toolbox  SourceProductBaseCode=RO
  Get Parameter2 : robotlib/Get Parameter  SourceLibraryInfo=This block requires Robotics System Toolbox  ParameterSource=Specify your own  ParameterName=/ropod/ropod_4wheel_kinb_cntr_node/smart_wheels/max_current  ParameterType=double  ParameterMaxArrayLength=16  ParameterInitialValue=max_sw_current  SampleTime=Tsp  ShowErrorCodeOutput=on  ModelName=ROPOD_4Wheel_Tdistkinb_cntr  BlockId=ParamGet_ROPOD_4Wheel_Tdistkinb_cntr_2215
      settings: SourceProductName=Robotics System Toolbox  SourceProductBaseCode=RO
  Get Parameter3 : robotlib/Get Parameter  SourceLibraryInfo=This block requires Robotics System Toolbox  ParameterSource=Specify your own  ParameterName=/ropod/ropod_4wheel_kinb_cntr_node/smart_wheels/pivot_offs_sw2  ParameterType=double  ParameterMaxArrayLength=16  ParameterInitialValue=pivot_offs_sws(2)  SampleTime=Tsp  ShowErrorCodeOutput=on  ModelName=ROPOD_4Wheel_Tdistkinb_cntr  BlockId=ParamGet_ROPOD_4Wheel_Tdistkinb_cntr_2216
      settings: SourceProductName=Robotics System Toolbox  SourceProductBaseCode=RO
  Get Parameter4 : robotlib/Get Parameter  SourceLibraryInfo=This block requires Robotics System Toolbox  ParameterSource=Specify your own  ParameterName=/ropod/ropod_4wheel_kinb_cntr_node/smart_wheels/pivot_offs_sw3  ParameterType=double  ParameterMaxArrayLength=16  ParameterInitialValue=pivot_offs_sws(3)  SampleTime=Tsp  ShowErrorCodeOutput=on  ModelName=ROPOD_4Wheel_Tdistkinb_cntr  BlockId=ParamGet_ROPOD_4Wheel_Tdistkinb_cntr_2217
      settings: SourceProductName=Robotics System Toolbox  SourceProductBaseCode=RO
  Get Parameter5 : robotlib/Get Parameter  SourceLibraryInfo=This block requires Robotics System Toolbox  ParameterSource=Specify your own  ParameterName=/ropod/ropod_4wheel_kinb_cntr_node/smart_wheels/pivot_offs_sw4  ParameterType=double  ParameterMaxArrayLength=16  ParameterInitialValue=pivot_offs_sws(4)  SampleTime=Tsp  ShowErrorCodeOutput=on  ModelName=ROPOD_4Wheel_Tdistkinb_cntr  BlockId=ParamGet_ROPOD_4Wheel_Tdistkinb_cntr_2218
      settings: SourceProductName=Robotics System Toolbox  SourceProductBaseCode=RO
  Get Parameter6 : robotlib/Get Parameter  SourceLibraryInfo=This block requires Robotics System Toolbox  ParameterSource=Specify your own  ParameterName=/ropod/ropod_4wheel_kinb_cntr_node/smart_wheels/dvarphi_LPF_fhz  ParameterType=double  ParameterMaxArrayLength=16  ParameterInitialValue=LPF_fhz_dvarphi_meas  SampleTime=Tsp  ShowErrorCodeOutput=on  ModelName=ROPOD_4Wheel_Tdistkinb_cntr  BlockId=ParamGet_ROPOD_4Wheel_Tdistkinb_cntr_4048
      settings: SourceProductName=Robotics System Toolbox  SourceProductBaseCode=RO
  Get Parameter7 : robotlib/Get Parameter  SourceLibraryInfo=This block requires Robotics System Toolbox  ParameterSource=Specify your own  ParameterName=/smart_wheels/ddelta_LPF_fhz  ParameterType=double  ParameterMaxArrayLength=16  ParameterInitialValue=LPF_fhz_ddelta_meas  SampleTime=Tsp  ShowErrorCodeOutput=on  ModelName=ROPOD_4Wheel_Tdistkinb_cntr  BlockId=ParamGet_ROPOD_4Wheel_Tdistkinb_cntr_4050
      settings: SourceProductName=Robotics System Toolbox  SourceProductBaseCode=RO
  Terminator{,1..7} (8 alike) : Terminator
  sw_conf : Outport
  wires:
  Get Parameter/2 -> Terminator/1
  Get Parameter/1 -> Bus Creator/1  "enable"
  Bus Creator/1 -> sw_conf/1
  Get Parameter2/2 -> Terminator2/1
  Get Parameter2/1 -> Bus Creator/2  "max_current"
  Get Parameter1/1 -> Bus Creator/3  "pivot_offs_sw1"
  Get Parameter1/2 -> Terminator1/1
  Get Parameter3/2 -> Terminator3/1
  Get Parameter3/1 -> Bus Creator/4  "pivot_offs_sw2"
  Get Parameter4/2 -> Terminator4/1
  Get Parameter4/1 -> Bus Creator/5  "pivot_offs_sw3"
  Get Parameter5/2 -> Terminator5/1
  Get Parameter5/1 -> Bus Creator/6  "pivot_offs_sw4"
  Get Parameter6/1 -> Bus Creator/7  "dvarphi_LPF_fhz"
  Get Parameter6/2 -> Terminator6/1
  Get Parameter7/2 -> Terminator7/1
  Get Parameter7/1 -> Bus Creator/8  "ddelta_LPF_fhz"

== system ROPOD_4Wheel_Tdistkinb_cntr_hosp_platform/ROS base conf ==
  Bus Creator : BusCreator  Inputs=4
  Get Parameter : robotlib/Get Parameter  SourceLibraryInfo=This block requires Robotics System Toolbox  ParameterSource=Specify your own  ParameterName=/ropod/ropod_4wheel_kinb_cntr_node/base_conf/max_acc_xy  ParameterType=double  ParameterMaxArrayLength=16  ParameterInitialValue=max_ropod_acc_xy  SampleTime=Tsp  ShowErrorCodeOutput=on  ModelName=ROPOD_4Wheel_Tdistkinb_cntr  BlockId=ParamGet_ROPOD_4Wheel_Tdistkinb_cntr_2237
      settings: SourceProductName=Robotics System Toolbox  SourceProductBaseCode=RO
  Get Parameter1 : robotlib/Get Parameter  SourceLibraryInfo=This block requires Robotics System Toolbox  ParameterSource=Specify your own  ParameterName=/ropod/ropod_4wheel_kinb_cntr_node/base_conf/max_vel_xy  ParameterType=double  ParameterMaxArrayLength=16  ParameterInitialValue=max_ropod_vel_xy  SampleTime=Tsp  ShowErrorCodeOutput=on  ModelName=ROPOD_4Wheel_Tdistkinb_cntr  BlockId=ParamGet_ROPOD_4Wheel_Tdistkinb_cntr_2238
      settings: SourceProductName=Robotics System Toolbox  SourceProductBaseCode=RO
  Get Parameter2 : robotlib/Get Parameter  SourceLibraryInfo=This block requires Robotics System Toolbox  ParameterSource=Specify your own  ParameterName=/ropod/ropod_4wheel_kinb_cntr_node/base_conf/max_acc_theta  ParameterType=double  ParameterMaxArrayLength=16  ParameterInitialValue=max_ropod_acc_theta  SampleTime=Tsp  ShowErrorCodeOutput=on  ModelName=ROPOD_4Wheel_Tdistkinb_cntr  BlockId=ParamGet_ROPOD_4Wheel_Tdistkinb_cntr_2239
      settings: SourceProductName=Robotics System Toolbox  SourceProductBaseCode=RO
  Get Parameter3 : robotlib/Get Parameter  SourceLibraryInfo=This block requires Robotics System Toolbox  ParameterSource=Specify your own  ParameterName=/ropod/ropod_4wheel_kinb_cntr_node/base_conf/max_vel_theta  ParameterType=double  ParameterMaxArrayLength=16  ParameterInitialValue=max_ropod_vel_theta  SampleTime=Tsp  ShowErrorCodeOutput=on  ModelName=ROPOD_4Wheel_Tdistkinb_cntr  BlockId=ParamGet_ROPOD_4Wheel_Tdistkinb_cntr_2240
      settings: SourceProductName=Robotics System Toolbox  SourceProductBaseCode=RO
  Terminator{,1..3} (4 alike) : Terminator
  base_conf : Outport
  wires:
  Get Parameter/2 -> Terminator/1
  Get Parameter1/2 -> Terminator1/1
  Get Parameter/1 -> Bus Creator/2  "max_acc_xy"
  Get Parameter1/1 -> Bus Creator/1  "max_vel_xy"
  Bus Creator/1 -> base_conf/1
  Get Parameter2/2 -> Terminator2/1
  Get Parameter2/1 -> Bus Creator/4  "max_acc_theta"
  Get Parameter3/1 -> Bus Creator/3  "max_vel_theta"
  Get Parameter3/2 -> Terminator3/1

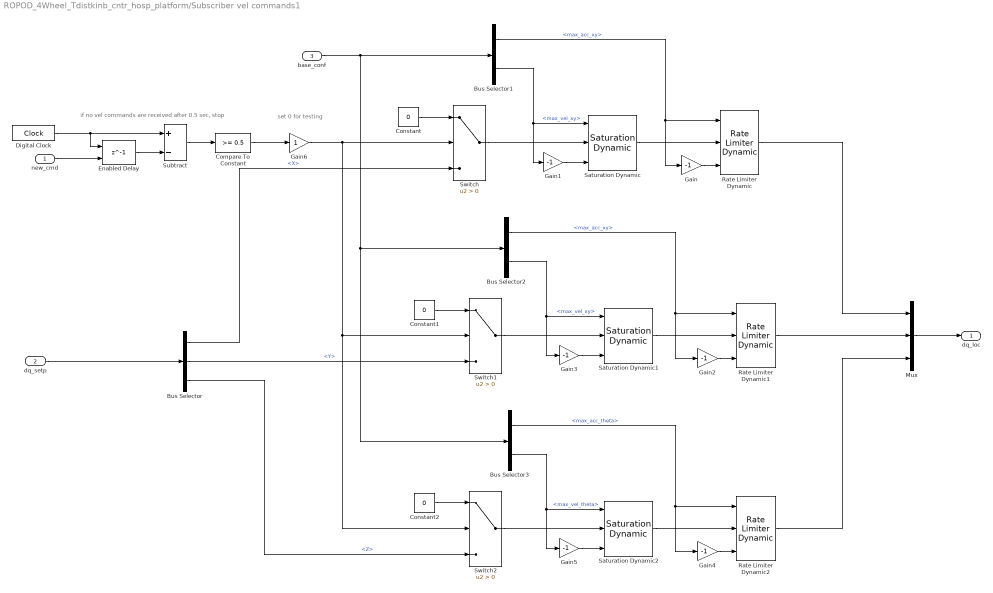
== system ROPOD_4Wheel_Tdistkinb_cntr_hosp_platform/Subscriber vel commands1 ==
  note: set 0 for testing
  note: if no vel commands are received after 0.5 sec, stop
  new_cmd : Inport
  dq_setp : Inport  Port=2
  base_conf : Inport  Port=3
  Bus Selector : BusSelector  OutputSignals=Linear.X,Linear.Y,Angular.Z
  Bus Selector1 : BusSelector  OutputSignals=max_acc_xy,max_vel_xy
  Bus Selector2 : BusSelector  OutputSignals=max_acc_xy,max_vel_xy
  Bus Selector3 : BusSelector  OutputSignals=max_acc_theta,max_vel_theta
  Compare To Constant : simulink/Logic and Bit Operations/Compare To Constant  relop=>=  const=0.5  OutDataTypeStr=boolean
  Constant : Constant  Value=0
  Constant1 : Constant  Value=0
  Constant2 : Constant  Value=0
  Digital Clock : DigitalClock
  Enabled Delay : Delay  DelayLength=1  ShowEnablePort=on
      settings: InputPortMap=u0,e6
  Gain{,1..5} (6 alike) : Gain  Gain=-1
  Gain6 : Gain
  Mux : Mux  Inputs=3
  Rate Limiter Dynamic : simulink/Discontinuities/Rate Limiter Dynamic
      settings: SourceProductName=Simulink
  Rate Limiter Dynamic1 : simulink/Discontinuities/Rate Limiter Dynamic
      settings: SourceProductName=Simulink
  Rate Limiter Dynamic2 : simulink/Discontinuities/Rate Limiter Dynamic
      settings: SourceProductName=Simulink
  Saturation Dynamic : simulink/Discontinuities/Saturation Dynamic  OutMin=[]  OutMax=[]  OutDataTypeStr=Inherit: Same as second input  OutDataType=fixdt(1, 16)  OutScaling=2^-10  DoSatur=off
  Saturation Dynamic1 : simulink/Discontinuities/Saturation Dynamic  OutMin=[]  OutMax=[]  OutDataTypeStr=Inherit: Same as second input  OutDataType=fixdt(1, 16)  OutScaling=2^-10  DoSatur=off
  Saturation Dynamic2 : simulink/Discontinuities/Saturation Dynamic  OutMin=[]  OutMax=[]  OutDataTypeStr=Inherit: Same as second input  OutDataType=fixdt(1, 16)  OutScaling=2^-10  DoSatur=off
  Subtract : Sum  Inputs=+-
  Switch : Switch  Criteria=u2 > Threshold
  Switch1 : Switch  Criteria=u2 > Threshold
  Switch2 : Switch  Criteria=u2 > Threshold
  dq_loc : Outport
  wires:
  Bus Selector/1 -> Switch/3  "<X>"
  dq_setp/1 -> Bus Selector/1
  new_cmd/1 -> Enabled Delay/2
  Digital Clock/1 -> Enabled Delay/1, Subtract/1
  Enabled Delay/1 -> Subtract/2
  Subtract/1 -> Compare To Constant/1
  Constant/1 -> Switch/1
  Gain/1 -> Rate Limiter Dynamic/3
  Switch/1 -> Saturation Dynamic/2
  Gain1/1 -> Saturation Dynamic/3
  Saturation Dynamic/1 -> Rate Limiter Dynamic/2
  Switch1/1 -> Saturation Dynamic1/2
  Gain3/1 -> Saturation Dynamic1/3
  Constant1/1 -> Switch1/1
  Bus Selector/2 -> Switch1/3  "<Y>"
  Gain2/1 -> Rate Limiter Dynamic1/3
  Saturation Dynamic1/1 -> Rate Limiter Dynamic1/2
  Bus Selector2/1 -> Rate Limiter Dynamic1/1, Gain2/1  "<max_acc_xy>"
  Bus Selector2/2 -> Saturation Dynamic1/1, Gain3/1  "<max_vel_xy>"
  Bus Selector3/1 -> Rate Limiter Dynamic2/1, Gain4/1  "<max_acc_theta>"
  Saturation Dynamic2/1 -> Rate Limiter Dynamic2/2
  base_conf/1 -> Bus Selector3/1, Bus Selector2/1, Bus Selector1/1
  Switch2/1 -> Saturation Dynamic2/2
  Constant2/1 -> Switch2/1
  Bus Selector/3 -> Switch2/3  "<Z>"
  Gain5/1 -> Saturation Dynamic2/3
  Gain4/1 -> Rate Limiter Dynamic2/3
  Compare To Constant/1 -> Gain6/1
  Bus Selector3/2 -> Saturation Dynamic2/1, Gain5/1  "<max_vel_theta>"
  Mux/1 -> dq_loc/1
  Rate Limiter Dynamic/1 -> Mux/1
  Rate Limiter Dynamic1/1 -> Mux/2
  Rate Limiter Dynamic2/1 -> Mux/3
  Bus Selector1/2 -> Saturation Dynamic/1, Gain1/1  "<max_vel_xy>"
  Bus Selector1/1 -> Rate Limiter Dynamic/1, Gain/1  "<max_acc_xy>"
  Gain6/1 -> Switch2/2, Switch1/2, Switch/2

== system ROPOD_4Wheel_Tdistkinb_cntr_hosp_platform/platform vel cntr ==
  ropod_kinmodel_pv : Inport
  sw_conf : Inport  Port=2
  disable : Inport  Port=3
  platform_dxdy_cntr_param : Inport  Port=4
  platform_dtheta_cntr_param : Inport  Port=5
  dqr_sp : Inport  Port=6
  dqr_loc : Inport  Port=7
  delta : Inport  Port=8
  ena_w : Inport  Port=9
  Inverse Kinematics 4SW : Subsystem
  Platorm Velocity controller : Subsystem
  Torque distribution : Subsystem
  dvarphi_sp : Outport
  varphi_tau_sp : Outport  Port=2
  wires:
  delta/1 -> Torque distribution/5(delta), Inverse Kinematics 4SW/3(delta)
  ena_w/1 -> Torque distribution/4(ena_w)
  sw_conf/1 -> Torque distribution/3(sw_conf)
  Torque distribution/1(varphi_tau_setp_out) -> varphi_tau_sp/1
  ropod_kinmodel_pv/1 -> Inverse Kinematics 4SW/1(param_in), Torque distribution/2(ropod_kinmodel_pv)
  Platorm Velocity controller/1(f_body_setp) -> Torque distribution/1(tau_body)
  disable/1 -> Platorm Velocity controller/1(reset_int)
  dqr_sp/1 -> Platorm Velocity controller/2(dqr_sp), Inverse Kinematics 4SW/2(dqr_sp)
  dqr_loc/1 -> Platorm Velocity controller/3(dqr_loc)
  Inverse Kinematics 4SW/1(wheel_vel_sp) -> dvarphi_sp/1
  platform_dxdy_cntr_param/1 -> Platorm Velocity controller/4(platform_dxdy_cntr_param)
  platform_dtheta_cntr_param/1 -> Platorm Velocity controller/5(platform_dtheta_cntr_param)

== system ROPOD_4Wheel_Tdistkinb_cntr_hosp_platform/wheel vel cntr ==
  disable : Inport
  platform_dxdy_cntr_param : Inport  Port=2
  dvarphi_sp : Inport  Port=3
  In5 : Inport  Port=4
  dvarphi : Inport  Port=5
  Sum : Sum  Inputs=-+|
  Wheels Velocity controller : Subsystem
  varphi_tau_setp_out : Outport
  wires:
  Wheels Velocity controller/1(varphi_tau_setp) -> varphi_tau_setp_out/1
  In5/1 -> Wheels Velocity controller/2(ena_w)
  Sum/1 -> Wheels Velocity controller/1(dvarphi_error)
  dvarphi/1 -> Sum/1
  dvarphi_sp/1 -> Sum/2
  disable/1 -> Wheels Velocity controller/4(reset_int)
  platform_dxdy_cntr_param/1 -> Wheels Velocity controller/3(platform_dvarphi_cntr_param)

== system ROPOD_4Wheel_Tdistkinb_cntr_hosp_platform/ROPOD 4SW TORQUE_MODE/Initialization switch ==
  vel_mode_enable : Inport
  In2 : Inport  Port=2
  Constant13 : Constant  Value=SW_COM1_MODE_TORQUE
  Constant5 : Constant  Value=SW_COM1_MODE_VELOCITY
  Movinf around SW axis center : Constant  Value=[2 -2 2 -2 2 -2 2 -2]
  Switch : Switch  Criteria=u2 ~= 0
  Switch1 : Switch  Criteria=u2 ~= 0
  cntr_mode : Outport
  wheel_setp : Outport  Port=2
  wires:
  Constant13/1 -> Switch/3
  Constant5/1 -> Switch/1
  vel_mode_enable/1 -> Switch/2, Switch1/2
  Switch1/1 -> wheel_setp/1
  Switch/1 -> cntr_mode/1
  Movinf around SW axis center/1 -> Switch1/1
  In2/1 -> Switch1/3

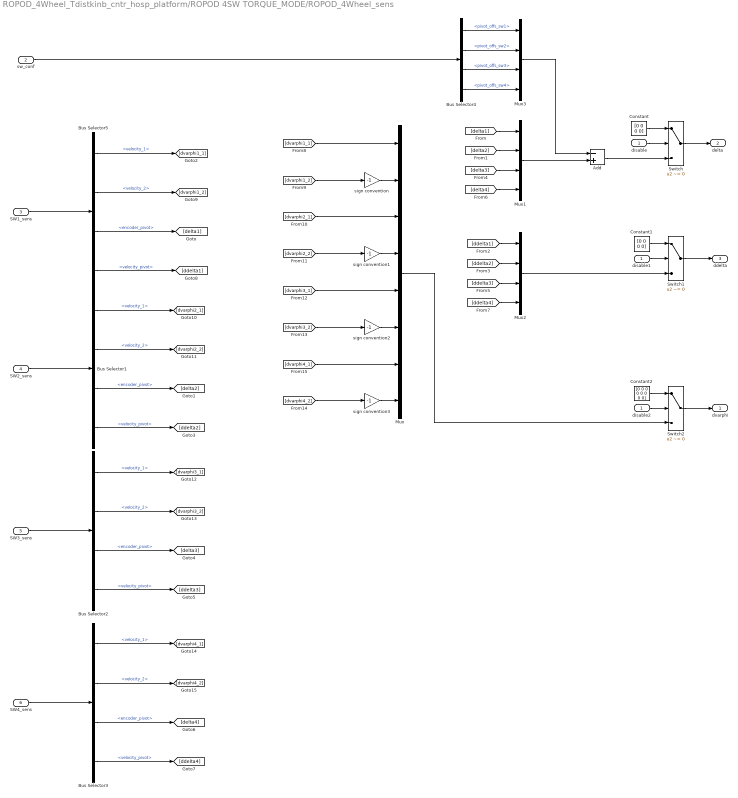
== system ROPOD_4Wheel_Tdistkinb_cntr_hosp_platform/ROPOD 4SW TORQUE_MODE/ROPOD_4Wheel_sens ==
  disable : Inport
  sw_conf : Inport  Port=2
  SW1_sens : Inport  Port=3
  SW2_sens : Inport  Port=4
  SW3_sens : Inport  Port=5
  SW4_sens : Inport  Port=6
  Add : Sum  Inputs=-+
  Bus Selector{1..3,5} (4 alike) : BusSelector  OutputSignals=velocity_1,velocity_2,encoder_pivot,velocity_pivot
  Bus Selector4 : BusSelector  OutputSignals=pivot_offs_sw1,pivot_offs_sw2,pivot_offs_sw3,pivot_offs_sw4
  Constant : Constant  Value=[0 0 0 0]
  Constant1 : Constant  Value=[0 0 0 0]
  Constant2 : Constant  Value=[0 0 0 0 0 0 0 0]
  Mux : Mux  Inputs=8
  Mux1 : Mux
  Mux2 : Mux
  Mux3 : Mux
  Switch : Switch  Criteria=u2 ~= 0
  Switch1 : Switch  Criteria=u2 ~= 0
  Switch2 : Switch  Criteria=u2 ~= 0
  disable1 : InportShadow
  disable2 : InportShadow
  sign convention{,1..3} (4 alike) : Gain  Gain=-1
  dvarphi : Outport
  delta : Outport  Port=2
  ddelta : Outport  Port=3
  wires:
  SW1_sens/1 -> Bus Selector5/1
  [delta1] -> Mux1/1
  [delta2] -> Mux1/2
  [ddelta2] -> Mux2/2
  [ddelta1] -> Mux2/1
  [delta3] -> Mux1/3
  [ddelta3] -> Mux2/3
  [delta4] -> Mux1/4
  [ddelta4] -> Mux2/4
  Mux1/1 -> Add/2
  Mux3/1 -> Add/1
  Bus Selector4/1 -> Mux3/1  "<pivot_offs_sw1>"
  Bus Selector4/2 -> Mux3/2  "<pivot_offs_sw2>"
  Bus Selector4/3 -> Mux3/3  "<pivot_offs_sw3>"
  Bus Selector4/4 -> Mux3/4  "<pivot_offs_sw4>"
  sign convention/1 -> Mux/2
  sign convention1/1 -> Mux/4
  sign convention2/1 -> Mux/6
  sign convention3/1 -> Mux/8
  Add/1 -> Switch/3
  Switch/1 -> delta/1
  disable/1 -> Switch/2
  Constant/1 -> Switch/1
  Switch1/1 -> ddelta/1
  Mux2/1 -> Switch1/3
  Constant1/1 -> Switch1/1
  disable1/1 -> Switch1/2
  disable2/1 -> Switch2/2
  Constant2/1 -> Switch2/1
  Mux/1 -> Switch2/3
  Switch2/1 -> dvarphi/1
  Bus Selector5/4 -> [ddelta1]  "<velocity_pivot>"
  Bus Selector5/2 -> [dvarphi1_2]  "<velocity_2>"
  sw_conf/1 -> Bus Selector4/1
  [dvarphi1_1] -> Mux/1
  [dvarphi1_2] -> sign convention/1
  [dvarphi2_1] -> Mux/3
  [dvarphi2_2] -> sign convention1/1
  [dvarphi3_1] -> Mux/5
  [dvarphi3_2] -> sign convention2/1
  [dvarphi4_1] -> Mux/7
  [dvarphi4_2] -> sign convention3/1
  Bus Selector5/1 -> [dvarphi1_1]  "<velocity_1>"
  Bus Selector5/3 -> [delta1]  "<encoder_pivot>"
  SW2_sens/1 -> Bus Selector1/1
  Bus Selector1/4 -> [ddelta2]  "<velocity_pivot>"
  Bus Selector1/1 -> [dvarphi2_1]  "<velocity_1>"
  Bus Selector1/3 -> [delta2]  "<encoder_pivot>"
  Bus Selector1/2 -> [dvarphi2_2]  "<velocity_2>"
  Bus Selector2/2 -> [dvarphi3_2]  "<velocity_2>"
  Bus Selector2/1 -> [dvarphi3_1]  "<velocity_1>"
  Bus Selector2/4 -> [ddelta3]  "<velocity_pivot>"
  SW3_sens/1 -> Bus Selector2/1
  Bus Selector2/3 -> [delta3]  "<encoder_pivot>"
  Bus Selector3/3 -> [delta4]  "<encoder_pivot>"
  SW4_sens/1 -> Bus Selector3/1
  Bus Selector3/4 -> [ddelta4]  "<velocity_pivot>"
  Bus Selector3/1 -> [dvarphi4_1]  "<velocity_1>"
  Bus Selector3/2 -> [dvarphi4_2]  "<velocity_2>"
